simulink model "FaultDetection"  (R2022b)
settings: configuration reference "BMS_Sw_CodeGenConfig" (kept outside this file)
libraries: FaultManagement_lib x8
settings Model: DataDictionary=Shared_DD.sldd  Creator=cpatel  LastModifiedBy=cpatel
settings ConfigSetRef: SourceName=BMS_Sw_CodeGenConfig

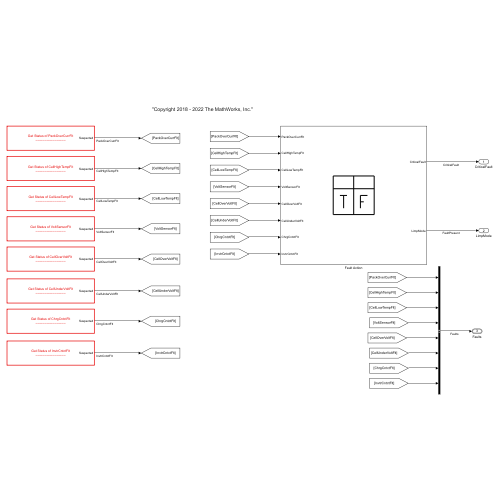
[thumbnail: Simulink's stored preview of the top-level diagram]
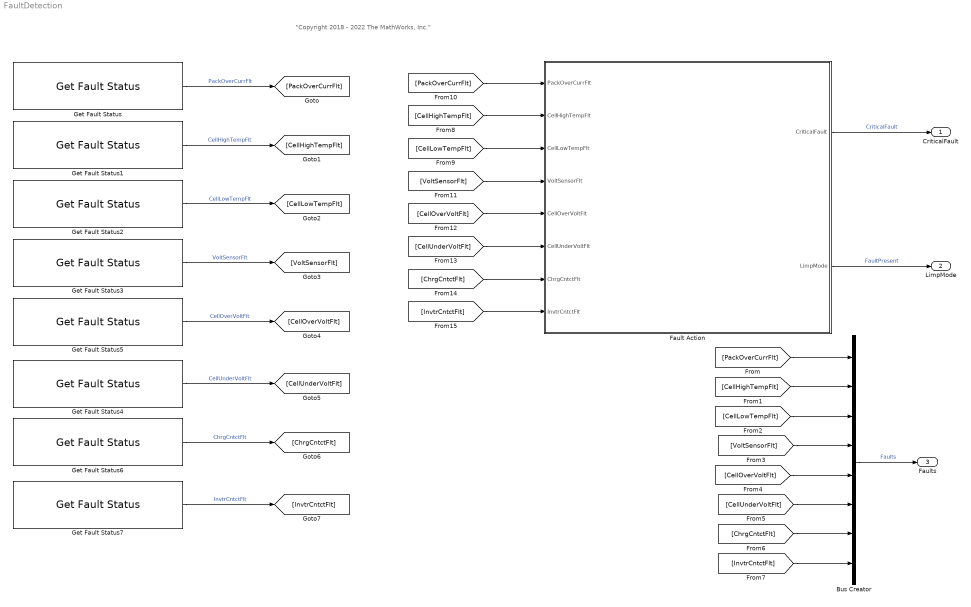
== system FaultDetection ==
  note: "Copyright 2018 - 2022 The MathWorks, Inc."
  Bus Creator : BusCreator  Inputs=8  OutDataTypeStr=Bus: Faults  NonVirtualBus=on
      settings: InheritFromInputs=off
  Fault Action : Truth Table  TreatAsAtomicUnit=on
  Get Fault Status : FaultManagement_lib/Get Fault Status  FaultName=PackOverCurrFlt  StatusField=Suspected
  Get Fault Status1 : FaultManagement_lib/Get Fault Status  FaultName=CellHighTempFlt  StatusField=Suspected
  Get Fault Status2 : FaultManagement_lib/Get Fault Status  FaultName=CellLowTempFlt  StatusField=Suspected
  Get Fault Status3 : FaultManagement_lib/Get Fault Status  FaultName=VoltSensorFlt  StatusField=Suspected
  Get Fault Status4 : FaultManagement_lib/Get Fault Status  FaultName=CellUnderVoltFlt  StatusField=Suspected
  Get Fault Status5 : FaultManagement_lib/Get Fault Status  FaultName=CellOverVoltFlt  StatusField=Suspected
  Get Fault Status6 : FaultManagement_lib/Get Fault Status  FaultName=ChrgCntctFlt  StatusField=Suspected
  Get Fault Status7 : FaultManagement_lib/Get Fault Status  FaultName=InvtrCntctFlt  StatusField=Suspected
  CriticalFault : Outport
  LimpMode : Outport  Port=2
  Faults : Outport  Port=3  OutDataTypeStr=Bus: Faults  VectorParamsAs1DForOutWhenUnconnected=off  BusOutputAsStruct=on
  wires:
  Bus Creator/1 -> Faults/1  "Faults"
  Fault Action/2(LimpMode) -> LimpMode/1  "FaultPresent"
  Get Fault Status/1 -> [PackOverCurrFlt]  "PackOverCurrFlt"
  Get Fault Status1/1 -> [CellHighTempFlt]  "CellHighTempFlt"
  Get Fault Status2/1 -> [CellLowTempFlt]  "CellLowTempFlt"
  Get Fault Status3/1 -> [VoltSensorFlt]  "VoltSensorFlt"
  Get Fault Status5/1 -> [CellOverVoltFlt]  "CellOverVoltFlt"
  Get Fault Status4/1 -> [CellUnderVoltFlt]  "CellUnderVoltFlt"
  Get Fault Status6/1 -> [ChrgCntctFlt]  "ChrgCntctFlt"
  Get Fault Status7/1 -> [InvtrCntctFlt]  "InvtrCntctFlt"
  [PackOverCurrFlt] -> Fault Action/1(PackOverCurrFlt)
  [PackOverCurrFlt] -> Bus Creator/1
  [CellHighTempFlt] -> Bus Creator/2
  [CellLowTempFlt] -> Bus Creator/3
  [VoltSensorFlt] -> Bus Creator/4
  [CellOverVoltFlt] -> Bus Creator/5
  [CellUnderVoltFlt] -> Bus Creator/6
  [ChrgCntctFlt] -> Bus Creator/7
  [InvtrCntctFlt] -> Bus Creator/8
  [CellHighTempFlt] -> Fault Action/2(CellHighTempFlt)
  [CellLowTempFlt] -> Fault Action/3(CellLowTempFlt)
  [VoltSensorFlt] -> Fault Action/4(VoltSensorFlt)
  [CellOverVoltFlt] -> Fault Action/5(CellOverVoltFlt)
  [CellUnderVoltFlt] -> Fault Action/6(CellUnderVoltFlt)
  [ChrgCntctFlt] -> Fault Action/7(ChrgCntctFlt)
  [InvtrCntctFlt] -> Fault Action/8(InvtrCntctFlt)
  Fault Action/1(CriticalFault) -> CriticalFault/1  "CriticalFault"

== matlab function FaultDetection/Fault Action ==
  data: PackOverCurrFlt input; CriticalFault output boolean size=1 =false; CellHighTempFlt input; CellLowTempFlt input; VoltSensorFlt input; CellOverVoltFlt input; CellUnderVoltFlt input; ChrgCntctFlt input; InvtrCntctFlt input; LimpMode output boolean =false
function [CriticalFault, LimpMode] = fcn(PackOverCurrFlt, CellHighTempFlt, CellLowTempFlt, VoltSensorFlt, CellOverVoltFlt, CellUnderVoltFlt, ChrgCntctFlt, InvtrCntctFlt)

aVarTruthTableCondition_1 = false;
aVarTruthTableCondition_2 = false;


% Any Non-Critical Fault Active

aVarTruthTableCondition_1 = logical(PackOverCurrFlt || CellHighTempFlt || CellLowTempFlt || CellOverVoltFlt || CellUnderVoltFlt ||   VoltSensorFlt);

% Critical Fault Active

aVarTruthTableCondition_2 = logical(ChrgCntctFlt || InvtrCntctFlt);

if (aVarTruthTableCondition_1)
    aFcnTruthTableAction_3();
elseif (aVarTruthTableCondition_2)
    aFcnTruthTableAction_2();
else % Default
    aFcnTruthTableAction_1();
end

function aFcnTruthTableAction_1()

% No Fault Not Present

CriticalFault = false;
LimpMode = false;

function aFcnTruthTableAction_2()

% Critical Fault Present

CriticalFault = true;

function aFcnTruthTableAction_3()

% Limp Mode Active

LimpMode = true;
